simulink model "directform2"  (R2022b)
settings: Solver=VariableStepAuto  StartTime=0.0  StopTime=1  RelTol=1e-3
libraries: spsFourierLib x2
settings Model: Creator=BURAK  LastModifiedBy=BURAK

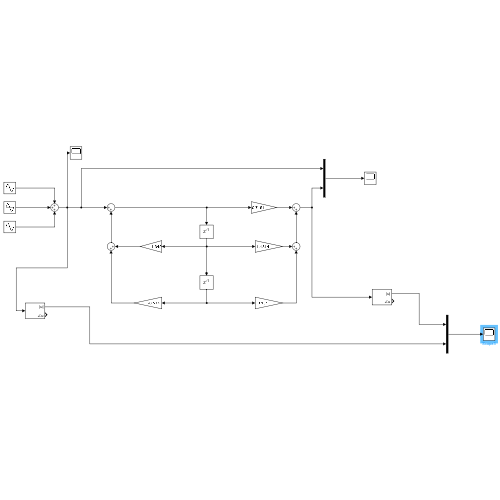
[thumbnail: Simulink's stored preview of the top-level diagram]
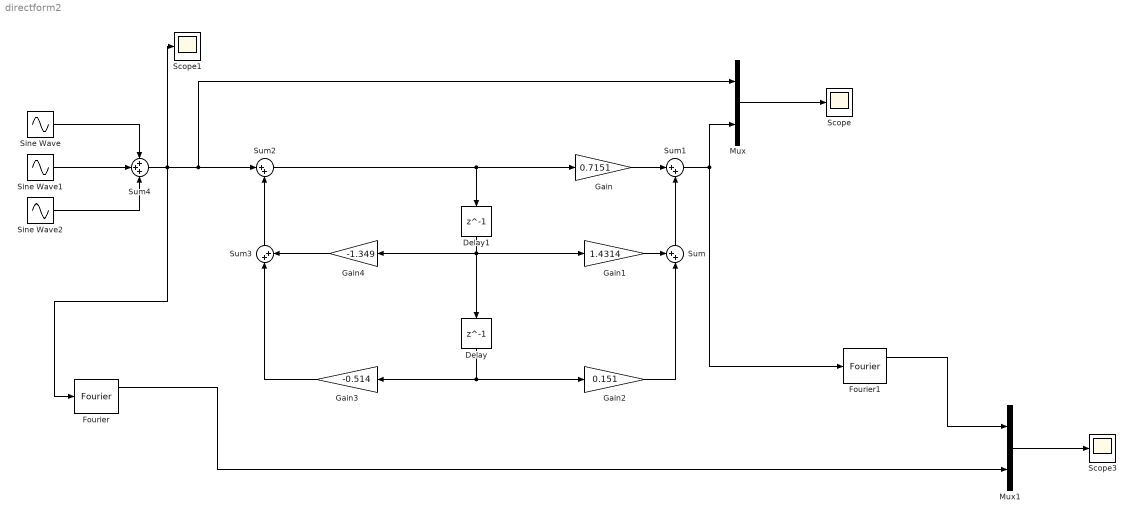
== system directform2 ==
  Delay : Delay  DelayLength=1  InitialCondition=0
  Delay1 : Delay  DelayLength=1  InitialCondition=0
  Fourier : spsFourierLib/Fourier  Freq=3  n=1  InInit=[0, 0]  Ts=0
  Fourier1 : spsFourierLib/Fourier  Freq=3  n=1  InInit=[0, 0]  Ts=0
  Gain : Gain  Gain=0.7151
  Gain1 : Gain  Gain=1.4314
  Gain2 : Gain  Gain=0.151
  Gain3 : Gain  Gain=-0.514
  Gain4 : Gain  Gain=-1.349
  Mux : Mux  Inputs=2
  Mux1 : Mux  Inputs=2
  Scope : Scope
  Scope1 : Scope
  Scope3 : Scope
  Sine Wave : Sin  Frequency=10  Phase=1.3  SampleTime=0
  Sine Wave1 : Sin  Frequency=20  SampleTime=0
  Sine Wave2 : Sin  Amplitude=2  Frequency=25  Phase=2.7  SampleTime=0
  Sum : Sum  Inputs=++|
  Sum1 : Sum  Inputs=|++
  Sum2 : Sum  Inputs=|++
  Sum3 : Sum  Inputs=|++
  Sum4 : Sum  Inputs=+++
  wires:
  Delay/1 -> Gain2/1, Gain3/1
  Delay1/1 -> Gain4/1, Delay/1, Gain1/1
  Gain1/1 -> Sum/1
  Gain2/1 -> Sum/2
  Gain/1 -> Sum1/1
  Sum/1 -> Sum1/2
  Gain4/1 -> Sum3/2
  Gain3/1 -> Sum3/1
  Sum3/1 -> Sum2/2
  Sum2/1 -> Gain/1, Delay1/1
  Mux/1 -> Scope/1
  Sum4/1 -> Fourier/1, Scope1/1, Mux/1, Sum2/1
  Sum1/1 -> Fourier1/1, Mux/2
  Fourier1/1 -> Mux1/1
  Fourier/1 -> Mux1/2
  Mux1/1 -> Scope3/1
  Sine Wave/1 -> Sum4/1
  Sine Wave1/1 -> Sum4/2
  Sine Wave2/1 -> Sum4/3
